simulink model "untitled"  (R2016a)
settings: Solver=VariableStepAuto  StartTime=0.0  StopTime=10.0  MaxStep=0.1  MinStep=0.01  RelTol=1e-3
undefined symbols (not defined in the file or in its folder): A0, A120, A150, A180, A30, A60, A90, B0, B120, B150, B180, B30, B60, B90
libraries: fuzblock x1
settings Model: Creator=student  LastModifiedBy=student

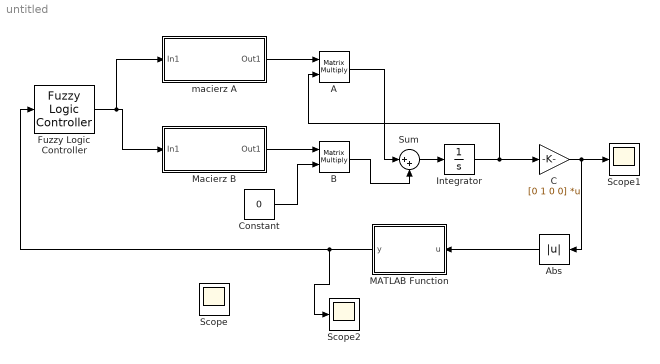
== system untitled ==
  A : Product  Multiplication=Matrix(*)
  Abs : Abs
  B : Product  Multiplication=Matrix(*)
  C : Gain  Gain=[0 1 0 0]  Multiplication=Matrix(K*u)
  Constant : Constant  Value=0
  Fuzzy Logic Controller : fuzblock/Fuzzy Logic  Controller  fis=['modelRozmyty.fis']
  Integrator : Integrator  InitialCondition=[0 pi 0 0]
  MATLAB Function : MATLAB Function  TreatAsAtomicUnit=on
  Macierz B : Subsystem
  Scope : Scope
  Scope1 : Scope
  Scope2 : Scope
  Sum : Sum  Inputs=|++
  "macierz A " : Subsystem
  wires:
  Fuzzy Logic Controller/1 -> "macierz A "/1(In1), Macierz B/1(In1)
  "macierz A "/1(Out1) -> A/1
  Macierz B/1(Out1) -> B/1
  B/1 -> Sum/2
  Sum/1 -> Integrator/1
  A/1 -> Sum/1
  Integrator/1 -> C/1, A/2
  Constant/1 -> B/2
  C/1 -> Abs/1, Scope1/1
  MATLAB Function/1(y) -> Scope2/1, Fuzzy Logic Controller/1
  Abs/1 -> MATLAB Function/1(u)

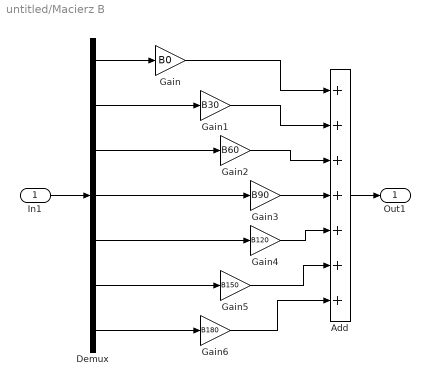
== system untitled/Macierz B ==
  In1 : Inport
  Add : Sum  Inputs=+++++++
  Demux : Demux  Outputs=7
  Gain : Gain  Gain=B0
  Gain1 : Gain  Gain=B30
  Gain2 : Gain  Gain=B60
  Gain3 : Gain  Gain=B90
  Gain4 : Gain  Gain=B120
  Gain5 : Gain  Gain=B150
  Gain6 : Gain  Gain=B180
  Out1 : Outport
  wires:
  In1/1 -> Demux/1
  Demux/2 -> Gain1/1
  Demux/3 -> Gain2/1
  Demux/1 -> Gain/1
  Demux/4 -> Gain3/1
  Demux/5 -> Gain4/1
  Demux/6 -> Gain5/1
  Demux/7 -> Gain6/1
  Gain/1 -> Add/1
  Gain1/1 -> Add/2
  Gain2/1 -> Add/3
  Gain3/1 -> Add/4
  Gain4/1 -> Add/5
  Gain5/1 -> Add/6
  Gain6/1 -> Add/7
  Add/1 -> Out1/1

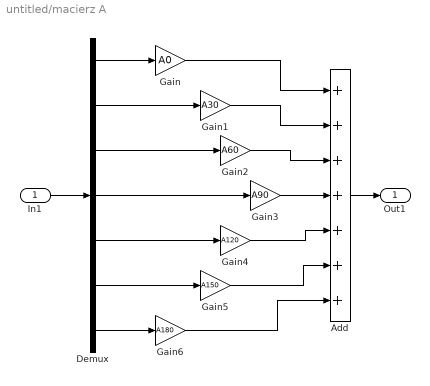
== system untitled/macierz A  ==
  In1 : Inport
  Add : Sum  Inputs=+++++++
  Demux : Demux  Outputs=7
  Gain : Gain  Gain=A0
  Gain1 : Gain  Gain=A30
  Gain2 : Gain  Gain=A60
  Gain3 : Gain  Gain=A90
  Gain4 : Gain  Gain=A120
  Gain5 : Gain  Gain=A150
  Gain6 : Gain  Gain=A180
  Out1 : Outport
  wires:
  In1/1 -> Demux/1
  Demux/2 -> Gain1/1
  Demux/3 -> Gain2/1
  Demux/1 -> Gain/1
  Demux/4 -> Gain3/1
  Demux/5 -> Gain4/1
  Demux/6 -> Gain5/1
  Demux/7 -> Gain6/1
  Gain/1 -> Add/1
  Gain1/1 -> Add/2
  Gain2/1 -> Add/3
  Gain3/1 -> Add/4
  Gain4/1 -> Add/5
  Gain5/1 -> Add/6
  Gain6/1 -> Add/7
  Add/1 -> Out1/1

== matlab function untitled/MATLAB Function ==
  data: u input; y output
function y = fcn(u)

g=u*pi/180;
if(u>180)
    reszta=rem(g,180);
    if(rem(fix(g/180),2)==1)
        g=180-reszta;
    else
        g=reszta;
    end

end
y = g;
